simulink model "HQEV_MiL_20160830_integrate"  (Simulink 8.3)
settings: Solver=FixedStepDiscrete  StartTime=0.0  StopTime=inf  FixedStep=0.01  RelTol=1e-3
PostLoadFcn:
  | , if any(exist('dsrtsu_mdlpostloadfcn', 'file') == [2, 3, 6]), try dsrtsu_mdlpostloadfcn('Execute', bdroot); catch fprintf('Error in PostLoadFcn (dsrtsu_mdlpostloadfcn) for model "%s":\n %s\n', bdroot, lasterr); end, end,
values from neighbouring files (symbols this model uses):
  Bat_C_Ah = 36    [parameter_V1.mat]
  Bat_ocv_xIndex = [5 10 20 30 40 50 60 70 80 90 95]    [parameter_V1.mat]
  Bat_ocv_z = [329 332 340 345 347 351 358 372 377 386 391]    [parameter_V1.mat]
  Bat_R_ohm_z = [4.41 3.46 1.57 1.07 0.76 0.63 0.55 0.44 0.41 0.4 0.4 3.14 ... (66 elements, 11x6)]    [parameter_V1.mat]
  Bat_SOC_Init = 90    [parameter_V1.mat]
  Env_hum_pct_Ambient = 30    [parameter_V1.mat]
  Env_Slope_deg = 0    [parameter_V1.mat]
  Env_Temp_degC_Ambient = 25    [parameter_V1.mat]
  Env_v_kmph_HWind = 0    [parameter_V1.mat]
  Reducer_F_i = 7.23    [parameter_V1.mat]
  Reducer_R_i = 7.23    [parameter_V1.mat]
  Veh =     [parameter_V1.mat]
  Veh_A_m2_Fr = 2.246    [parameter_V1.mat]
  Veh_F_Brake =     [parameter_V1.mat]
  Veh_fac_AirDrag = 0.326    [parameter_V1.mat]
  Veh_fac_WhDragFrict_0 = 0.011    [parameter_V1.mat]
  Veh_g_mps2_C = 9.81    [parameter_V1.mat]
  Veh_GainBrake =     [parameter_V1.mat]
  Veh_h_m_COGHigh = 0.5    [parameter_V1.mat]
  Veh_J_kgm2_Wh = 1.3635    [parameter_V1.mat]
  Veh_L_m_AxlBas = 2.63    [parameter_V1.mat]
  Veh_M_kg = 1427    [parameter_V1.mat]
  Veh_mu_Brake = 0.4    [parameter_V1.mat]
  Veh_mu_Tyre =     [parameter_V1.mat]
  Veh_num_FrictPair = 8    [parameter_V1.mat]
  Veh_pct_Brk = 70    [parameter_V1.mat]
  Veh_r_dyn =     [parameter_V1.mat]
  Veh_r_m_BrkDisk = 0.136    [parameter_V1.mat]
  Veh_rho_kgpm3_Air = 1.2258    [parameter_V1.mat]
undefined symbols (not defined in the file or in its folder): DiscIntNeverNeededParam, p_bool_False_M, p_bool_True_M
libraries: BaseOperationLib_Browser x38, simulink x9, DTQC_lib x1, ERR_lib x1, MQM_lib x1, PTCL_lib x1, PUD_lib x1, TQD_lib x1, TQR_lib x1, VMM_lib x1, ACCA_lib x1, BBCA_lib x1
(part 8 of 15)

== system HQEV_MiL_20160830_integrate/MiL/Test_Integration/DCDC/DCDC/DCDC/Electric_Manage ==
  DCDC_enable : Inport
  V_out_req : Inport  Port=2
  Battery_Voltage : Inport  Port=3
  IO_In1 : Inport  Port=4
  Constant1 : Constant  Value=0
  Constant2 : Constant  Value=400
  Constant4 : Constant  Value=0.85
  DCDCStatus : Subsystem
  Divide : Product  Inputs=*/
  Divide1 : Product  Inputs=*/
  Multiport Switch : MultiPortSwitch  DataPortOrder=Zero-based contiguous  Inputs=2  zeroidx=on
  P/U : Product  Inputs=*/
  Saturation : Saturate  UpperLimit=30  LowerLimit=10
  Saturation1 : Saturate  UpperLimit=500  LowerLimit=200
  DCDC_Status : Outport
  DCDC_pwr_Output : Outport  Port=2
  DCDC_pwr_Input : Outport  Port=3
  DCDC_I_Input : Outport  Port=4
  DCDC_U_Input : Outport  Port=5
  DCDC_I_Output : Outport  Port=6
  DCDC_U_Output : Outport  Port=7
  wires:
  V_out_req/1 -> Saturation/1
  P/U/1 -> DCDC_I_Output/1
  DCDC_enable/1 -> Multiport Switch/1, DCDCStatus/1(DCDC_Enable)
  Multiport Switch/1 -> P/U/1, Divide/1, DCDC_pwr_Output/1
  Constant1/1 -> Multiport Switch/2
  Saturation/1 -> P/U/2, DCDC_U_Output/1
  Constant4/1 -> Divide/2
  Battery_Voltage/1 -> Saturation1/1
  Saturation1/1 -> Divide1/2, DCDC_U_Input/1
  Divide1/1 -> DCDC_I_Input/1
  DCDCStatus/1(StatusDCDC) -> DCDC_Status/1
  Divide/1 -> Divide1/1, DCDC_pwr_Input/1
  Constant2/1 -> Multiport Switch/3
  IO_In1/1 -> DCDCStatus/2(IO_In1)

== system HQEV_MiL_20160830_integrate/MiL/Test_Integration/DCDC/DCDC/Output/Checksum_DCDC1 ==
  In1 : Inport
  Constant : Constant  Value=0
  Terminator : Terminator
  Checksum_DCDC1 : Outport
  wires:
  Constant/1 -> Checksum_DCDC1/1
  In1/1 -> Terminator/1

== system HQEV_MiL_20160830_integrate/MiL/Test_Integration/DCDC/DCDC/Output/DCDCLoss ==
  In1 : Inport
  Bus Selector : BusSelector  OutputSignals=signal2.DCDC_Input_Power
  Constant : Constant  Value=0.15
  Product : Product  RndMeth=Zero
  pwr_DCDCLoss : Outport
  wires:
  Bus Selector/1 -> Product/1  "<DCDC_Input_Power>"
  In1/1 -> Bus Selector/1
  Constant/1 -> Product/2
  Product/1 -> pwr_DCDCLoss/1

== system HQEV_MiL_20160830_integrate/MiL/Test_Integration/DCDC/DCDC/Output/DCDC_InputCurrent ==
  In1 : Inport
  Bus Selector : BusSelector  OutputSignals=signal2.DCDC_Input_Current
  DCDC_in_Current : Outport
  wires:
  In1/1 -> Bus Selector/1
  Bus Selector/1 -> DCDC_in_Current/1  "<DCDC_Input_Current>"

== system HQEV_MiL_20160830_integrate/MiL/Test_Integration/DCDC/DCDC/Output/DCDC_InputVoltage ==
  In1 : Inport
  Bus Selector : BusSelector  OutputSignals=signal2.DCDC_Input_Voltage
  DCDC_Input_Voltage : Outport
  wires:
  In1/1 -> Bus Selector/1
  Bus Selector/1 -> DCDC_Input_Voltage/1  "<DCDC_Input_Voltage>"

== system HQEV_MiL_20160830_integrate/MiL/Test_Integration/DCDC/DCDC/Output/DCDC_Input_Powr ==
  In1 : Inport
  Bus Selector : BusSelector  OutputSignals=signal2.DCDC_Input_Power
  DCDC_Input_Power : Outport
  wires:
  In1/1 -> Bus Selector/1
  Bus Selector/1 -> DCDC_Input_Power/1  "<DCDC_Input_Power>"

== system HQEV_MiL_20160830_integrate/MiL/Test_Integration/DCDC/DCDC/Output/DCDC_OutputCurrent ==
  In : Inport
  Bus Selector : BusSelector  OutputSignals=signal2.DCDC_Output_Current
  DCDC_Output_Current : Outport
  wires:
  Bus Selector/1 -> DCDC_Output_Current/1  "<DCDC_Output_Current>"
  In/1 -> Bus Selector/1

== system HQEV_MiL_20160830_integrate/MiL/Test_Integration/DCDC/DCDC/Output/DCDC_OutputVoltage ==
  In1 : Inport
  Bus Selector : BusSelector  OutputSignals=signal2.DCDC_Output_Voltage
  DCDC_Output_Voltage : Outport
  wires:
  In1/1 -> Bus Selector/1
  Bus Selector/1 -> DCDC_Output_Voltage/1  "<DCDC_Output_Voltage>"

== system HQEV_MiL_20160830_integrate/MiL/Test_Integration/DCDC/DCDC/Output/DCDC_Status ==
  In1 : Inport
  Bus Selector : BusSelector  OutputSignals=signal2.DCDC_Status
  DCDC_Status : Outport
  wires:
  In1/1 -> Bus Selector/1
  Bus Selector/1 -> DCDC_Status/1  "<DCDC_Status>"

== system HQEV_MiL_20160830_integrate/MiL/Test_Integration/DCDC/DCDC/Output/DCDC_Temperature ==
  Constant : Constant  Value=30
  DCDC_Temperature : Outport
  wires:
  Constant/1 -> DCDC_Temperature/1

== system HQEV_MiL_20160830_integrate/MiL/Test_Integration/DCDC/DCDC/Output/LiveCounter_DCDC_1 ==
  In1 : Inport
  Constant : Constant  Value=0
  Terminator : Terminator
  LiveCounter_DCDC1 : Outport
  wires:
  In1/1 -> Terminator/1
  Constant/1 -> LiveCounter_DCDC1/1

== system HQEV_MiL_20160830_integrate/MiL/Test_Integration/Driver/Driver/Control_Panel/ACButton ==
  note: 0 no press
      | 1      press
  IO_IN : Inport
  Bus Selector : BusSelector  OutputSignals=AC_Button
  out : Outport
  wires:
  Bus Selector/1 -> out/1  "<AC_Button>"
  IO_IN/1 -> Bus Selector/1

== system HQEV_MiL_20160830_integrate/MiL/Test_Integration/Driver/Driver/Control_Panel/ACC_Cruise_Button ==
  IO_IN : Inport
  Bus Selector : BusSelector  OutputSignals=ACCCruseInput
  Cancel_2 : Constant  Value=1000
  Error : Constant  Value=10000
  Headway_4 : Constant  Value=3200
  MainOff_0 : Constant  Value=5000
  MainOn_1 : Constant  Value=4500
  Multiport Switch : MultiPortSwitch  DataPortOrder=Zero-based contiguous  Inputs=7  zeroidx=on
  Resume_5 : Constant  Value=3900
  Set_3 : Constant  Value=2300
  out : Outport
  wires:
  IO_IN/1 -> Bus Selector/1
  Bus Selector/1 -> Multiport Switch/1  "<ACCCruseInput>"
  MainOff_0/1 -> Multiport Switch/2
  MainOn_1/1 -> Multiport Switch/3
  Cancel_2/1 -> Multiport Switch/4
  Set_3/1 -> Multiport Switch/5
  Headway_4/1 -> Multiport Switch/6
  Resume_5/1 -> Multiport Switch/7
  Multiport Switch/1 -> out/1
  Error/1 -> Multiport Switch/8

== system HQEV_MiL_20160830_integrate/MiL/Test_Integration/Driver/Driver/Control_Panel/ACStation_U ==
  Constant : Constant  Value=220
  out : Outport
  wires:
  Constant/1 -> out/1

== system HQEV_MiL_20160830_integrate/MiL/Test_Integration/Driver/Driver/Control_Panel/CP ==
  Constant : Constant  Value=0
  out : Outport
  wires:
  Constant/1 -> out/1

== system HQEV_MiL_20160830_integrate/MiL/Test_Integration/Driver/Driver/Control_Panel/EGSM_ECOSButton ==
  note: 0 no press
      | 1      press
  Constant : Constant  Value=0
  out : Outport
  wires:
  Constant/1 -> out/1

== system HQEV_MiL_20160830_integrate/MiL/Test_Integration/Driver/Driver/Control_Panel/EGSM_KnobPosition ==
  note: 0  center
      | 1        up
      | 3   down
  Constant : Constant  Value=0
  out : Outport
  wires:
  Constant/1 -> out/1

== system HQEV_MiL_20160830_integrate/MiL/Test_Integration/Driver/Driver/Control_Panel/EGSM_ParkButton ==
  note: 0 no press
      | 1      press
  Constant : Constant  Value=0
  out : Outport
  wires:
  Constant/1 -> out/1

== system HQEV_MiL_20160830_integrate/MiL/Test_Integration/Driver/Driver/Control_Panel/EGSM_SecurityButton ==
  note: 0 no press
      | 1      press
  Constant : Constant  Value=0
  out : Outport
  wires:
  Constant/1 -> out/1

== system HQEV_MiL_20160830_integrate/MiL/Test_Integration/Driver/Driver/Control_Panel/FastCharge ==
  IO_IN : Inport
  Bus Selector : BusSelector  OutputSignals=ChargeCheck
  ChargeFault : Constant  Value=220
  FastCharge : Constant  Value=1020
  Multiport Switch : MultiPortSwitch  DataPortOrder=Zero-based contiguous  Inputs=4  zeroidx=on
  NoCharge : Constant  Value=0
  Saturation : Saturate  UpperLimit=3  LowerLimit=0
  SlowCharge : Constant  Value=270
  out : Outport
  wires:
  Bus Selector/1 -> Saturation/1  "<ChargeCheck>"
  IO_IN/1 -> Bus Selector/1
  Multiport Switch/1 -> out/1
  NoCharge/1 -> Multiport Switch/2
  ChargeFault/1 -> Multiport Switch/5
  Saturation/1 -> Multiport Switch/1
  SlowCharge/1 -> Multiport Switch/4
  FastCharge/1 -> Multiport Switch/3

== system HQEV_MiL_20160830_integrate/MiL/Test_Integration/Driver/Driver/Control_Panel/InterlockA ==
  IO_IN : Inport
  Bus Selector : BusSelector  OutputSignals=interlockA
  Compare To Constant : simulink/Logic and Bit Operations/Compare To Constant  SystemSampleTime=-1  relop===  const=0  LogicOutDataTypeMode=boolean
  Init : Constant  Value=2500
  Switch : Switch  Criteria=u2 > Threshold
  out : Outport
  wires:
  IO_IN/1 -> Bus Selector/1
  Bus Selector/1 -> Switch/3, Compare To Constant/1  "<interlockA>"
  Compare To Constant/1 -> Switch/2
  Init/1 -> Switch/1
  Switch/1 -> out/1

== system HQEV_MiL_20160830_integrate/MiL/Test_Integration/Driver/Driver/Control_Panel/InterlockB ==
  IO_IN : Inport
  Bus Selector : BusSelector  OutputSignals=interlockB
  Compare To Constant : simulink/Logic and Bit Operations/Compare To Constant  SystemSampleTime=-1  relop===  const=0  LogicOutDataTypeMode=boolean
  Init : Constant  Value=2500
  Switch : Switch  Criteria=u2 > Threshold
  out : Outport
  wires:
  IO_IN/1 -> Bus Selector/1
  Compare To Constant/1 -> Switch/2
  Init/1 -> Switch/1
  Bus Selector/1 -> Switch/3, Compare To Constant/1  "<interlockB>"
  Switch/1 -> out/1

== system HQEV_MiL_20160830_integrate/MiL/Test_Integration/Driver/Driver/Control_Panel/KeyONState ==
  IO_IN : Inport
  Bus Selector : BusSelector  OutputSignals=KeyOn
  out : Outport
  wires:
  Bus Selector/1 -> out/1  "<KeyOn>"
  IO_IN/1 -> Bus Selector/1

== system HQEV_MiL_20160830_integrate/MiL/Test_Integration/Driver/Driver/Control_Panel/KeyStartState ==
  IO_IN : Inport
  Bus Selector : BusSelector  OutputSignals=KeyStart
  out : Outport
  wires:
  Bus Selector/1 -> out/1  "<KeyStart>"
  IO_IN/1 -> Bus Selector/1

== system HQEV_MiL_20160830_integrate/MiL/Test_Integration/Driver/Driver/Control_Panel/LeverPosition ==
  note: 0--Center
      | 1--up
      | 2--down
      | 3--up up
      | 4--down down
  IO_IN : Inport
  Bus Selector : BusSelector  OutputSignals=ShiftLeverInput
  Center : Constant  Value=0
  Down : Constant  Value=2
  DownDown : Constant  Value=4
  Multiport Switch : MultiPortSwitch  DataPortOrder=Zero-based contiguous  Inputs=5  zeroidx=on
  Saturation : Saturate  UpperLimit=4  LowerLimit=0
  Up : Constant
  UpUp : Constant  Value=3
  out : Outport
  wires:
  Multiport Switch/1 -> out/1
  IO_IN/1 -> Bus Selector/1
  Bus Selector/1 -> Saturation/1  "<ShiftLeverInput>"
  Center/1 -> Multiport Switch/2
  Up/1 -> Multiport Switch/3
  Down/1 -> Multiport Switch/4
  UpUp/1 -> Multiport Switch/5
  DownDown/1 -> Multiport Switch/6
  Saturation/1 -> Multiport Switch/1

== system HQEV_MiL_20160830_integrate/MiL/Test_Integration/Driver/Driver/Control_Panel/RunSignal ==
  Constant : Constant  Value=0
  out : Outport
  wires:
  Constant/1 -> out/1

== system HQEV_MiL_20160830_integrate/MiL/Test_Integration/Driver/Driver/Driver_AutoPedal/CTRL AccPed ==
  v_set [km/h] : Inport
  v_Veh [km/h] : Inport  Port=2
  Brake [%] : Inport  Port=3
  Brake off : Subsystem  mask(Compare To Constant){relop=<=, const=eps, LogicOutDataTypeMode=uint8, ZeroCross=off}
      mask prompts: relop "Operator:"; const "Constant value:"; LogicOutDataTypeMode "Output data type mode:"; ZeroCross "Enable zero crossing detection"
      mask help: Determine how a signal compares to a constant.
      mask init:
      | blkName = gcb;
      | 
      | if strcmp(get_param(gcbh,'LogicOutDataTypeMode'),'boolean')
      | 	setValue = 'Boolean';
      | else
      | 	setValue = 'Specify via dialog';
      | end
      | 
      | set_param([blkName,'/Compare'],'relop',relop, ...
      | 	'LogicOutDataTypeMode', setValue, 'ZeroCross', ZeroCross);
      | 
      | str = [relop,' C']; %default
      | 
      | const_str = get_param(blkName, 'const');
      | 
      | if isempty(strfind(const_str, ' ')) && isempty(strfind(const_str, ','))
      |     % scalar or single expression
      |     if isempty(str2num(const_str))
      |         %expression
      |         str = [relop, ' ', const_str];
      |     elseif length(const) == 1
      |         str = [relop,' ',num2str(double(const))];
      |     end
      | end
      mask TypeOptions relop: == | ~= | < | <= | >= | >
      mask TypeOptions LogicOutDataTypeMode: uint8 | boolean
      mask Callback ZeroCross: sl('zeroCrossEnable', gcbh);
      mask Display: disp(str)
  Constant : Constant  Value=0
  Constant4 : Constant  Value=0
  Discrete-Time Integrator : DiscreteIntegrator  ExternalReset=rising  InitialConditionSource=external  SampleTime=-1  LimitOutput=on  UpperSaturationLimit=50  LowerSaturationLimit=-20  ICPrevOutput=DiscIntNeverNeededParam  ICPrevScaledInput=DiscIntNeverNeededParam
  I_value : Gain  Gain=0.1  SaturateOnIntegerOverflow=on  OutDataTypeStr=Inherit: Same as input  ParamDataTypeStr=Inherit: Same as input
  P_value : Gain  Gain=0.1  SaturateOnIntegerOverflow=on  OutDataTypeStr=Inherit: Same as input  ParamDataTypeStr=Inherit: Same as input
  Reset : Subsystem
  Saturation : Saturate  UpperLimit=100  LowerLimit=0
  Subsystem : Subsystem
  Sum : Sum  Inputs=|++  SaturateOnIntegerOverflow=on  InputSameDT=on  OutDataTypeStr=Inherit: Same as first input
  Switch3 : Switch  Criteria=u2 ~= 0  Threshold=0.5
  Sig_AccPed [%] : Outport
  wires:
  Subsystem/1(error) -> I_value/1, Reset/1(v_error), P_value/1
  Constant/1 -> Discrete-Time Integrator/3
  I_value/1 -> Discrete-Time Integrator/1
  Reset/1(reset) -> Discrete-Time Integrator/2
  P_value/1 -> Sum/1  "P-Anteil"
  Discrete-Time Integrator/1 -> Sum/2  "I-Anteil"
  Saturation/1 -> Switch3/1  "Gaspedal"
  Brake off/1(y) -> Switch3/2
  Sum/1 -> Saturation/1  "result"
  Constant4/1 -> Switch3/3
  Switch3/1 -> Sig_AccPed [%]/1
  Brake [%]/1 -> Reset/3(Brake [%]), Brake off/1(u)
  v_set [km/h]/1 -> Subsystem/1(v_Set), Reset/2(v_Set)
  v_Veh [km/h]/1 -> Subsystem/2(v_Veh)

== system HQEV_MiL_20160830_integrate/MiL/Test_Integration/Driver/Driver/Driver_AutoPedal/CTRL BrakePed ==
  v_set [km/h] : Inport
  v_Veh [km/h] : Inport  Port=2
  Bus Creator : BusCreator  Inputs=6
  Bus Selector : BusSelector  OutputSignals=v_set,v_Veh
  Bus Selector1 : BusSelector  OutputSignals=delta_v_set,v_error
  Bus Selector2 : BusSelector  OutputSignals=delta_v_set,v_error,v_Veh,Brake,Brake_set
  Bus Selector3 : BusSelector  OutputSignals=v_error
  Bus Selector4 : BusSelector  OutputSignals=v_set
  Constant : Constant  Value=50
  PI-Regler : Subsystem
  Reset_Block : Subsystem
  S-R Flip-Flop : Subsystem  mask(SRFlipFlop){initial_condition=0}
      mask prompts: initial_condition "Initial condition (state of Q):"
      mask help: S-R Flip-Flop Block
      mask Help:
      | The S-R flip-flop also known as a set-reset flip-flop. This implementation
      | is modeled after an S-R flip-flop constructed using NOR gates. The
      | truth table for this block is:
      | <pre>
      |  S  R   Q  !Q
      |  ----------------
      |  1  0   1  0
      |  0  0   1  0  (after S == 1, R == 0)
      |  0  1   0  1
      |  0  0   0  1  (after S == 0, R == 1)
      |  1  1   0  0
      | </pre>
      | 
      | In an S-R flip-flop that is implemented with NOR gates, when a 1 is
      | applied to both the set and reset inputs, both outputs go to 0. Technically,
      | this state is undefined and is usually avoided. Note, if the flip-flop is
      | implemented with NAND gates, when a 0 is applied to both inputs, both outputs
      | go to 0 and when a 1 is applied to both inputs, the output depends on
      | the previous state of the flip-flop (previous value of Q).
  Set_Block : Subsystem
  Switch : Switch  Criteria=u2 > Threshold
  Terminator : Terminator
  Unit Delay1 : UnitDelay  SampleTime=-1
  velocoty : Subsystem
  "Brake[%] " : Outport
  wires:
  PI-Regler/1(Result) -> Unit Delay1/1, Switch/1
  Reset_Block/1(Brake_Reset) -> S-R Flip-Flop/2(R)
  S-R Flip-Flop/2(!Q) -> Terminator/1
  S-R Flip-Flop/1(Q) -> PI-Regler/Enable
  Set_Block/1(Brake_set) -> S-R Flip-Flop/1(S), Bus Creator/3  "Brake_set"
  v_Veh [km/h]/1 -> Bus Creator/6  "v_Veh"
  v_set [km/h]/1 -> Bus Creator/5  "v_set"
  velocoty/1(delta_v_set) -> Bus Creator/1  "delta_v_set"
  velocoty/2(v_error) -> Bus Creator/2  "v_error"
  Unit Delay1/1 -> Bus Creator/4  "Brake"
  Bus Creator/1 -> Bus Selector/1, Bus Selector1/1, Bus Selector2/1, Bus Selector3/1, Bus Selector4/1
  Bus Selector/1 -> velocoty/1(v_set [km/h])  "<v_set>"
  Bus Selector/2 -> velocoty/2(v_Veh [km/h])  "<v_Veh>"
  Bus Selector1/1 -> Set_Block/1(delta_v_set)  "<delta_v_set>"
  Bus Selector1/2 -> Set_Block/2(v_error)  "<v_error>"
  Bus Selector2/1 -> Reset_Block/1(delta_v_set)  "<delta_v_set>"
  Bus Selector2/2 -> Reset_Block/2(v_error)  "<v_error>"
  Bus Selector2/3 -> Reset_Block/3(v_Veh)  "<v_Veh>"
  Bus Selector2/4 -> Reset_Block/4(Brake)  "<Brake>"
  Bus Selector2/5 -> Reset_Block/5(Brake_Set)  "<Brake_set>"
  Bus Selector3/1 -> PI-Regler/1(error)  "<v_error>"
  Bus Selector4/1 -> Switch/2  "<v_set>"
  Switch/1 -> "Brake[%] "/1
  Constant/1 -> Switch/3

== system HQEV_MiL_20160830_integrate/MiL/Test_Integration/Driver/Driver/Driver_AutoPedal/Stop_Indicator ==
  v_set : Inport
  Logical Operator : Logic  AllPortsSameDT=off  OutDataTypeStr=boolean
  Logical Operator1 : Logic  AllPortsSameDT=off  OutDataTypeStr=boolean
  Logical Operator2 : Logic  Operator=OR  AllPortsSameDT=off  OutDataTypeStr=boolean
  v_Set<0 : Subsystem  mask(Compare To Constant){relop=>=, const=-eps, LogicOutDataTypeMode=uint8, ZeroCross=off}
      mask prompts: relop "Operator:"; const "Constant value:"; LogicOutDataTypeMode "Output data type mode:"; ZeroCross "Enable zero crossing detection"
      mask help: Determine how a signal compares to a constant.
      mask init: same as HQEV_MiL_20160830_integrate/MiL/Test_Integration/Driver/Driver/Driver_AutoPedal/CTRL AccPed/Brake off
      mask TypeOptions relop: == | ~= | < | <= | >= | >
      mask TypeOptions LogicOutDataTypeMode: uint8 | boolean
      mask Callback ZeroCross: sl('zeroCrossEnable', gcbh);
      mask Display: disp(str)
  v_Set==1 : Subsystem  mask(Compare To Constant){relop=<, const=0, LogicOutDataTypeMode=uint8, ZeroCross=off}
      mask prompts: relop "Operator:"; const "Constant value:"; LogicOutDataTypeMode "Output data type mode:"; ZeroCross "Enable zero crossing detection"
      mask help: Determine how a signal compares to a constant.
      mask init: same as HQEV_MiL_20160830_integrate/MiL/Test_Integration/Driver/Driver/Driver_AutoPedal/CTRL AccPed/Brake off
      mask TypeOptions relop: == | ~= | < | <= | >= | >
      mask TypeOptions LogicOutDataTypeMode: uint8 | boolean
      mask Callback ZeroCross: sl('zeroCrossEnable', gcbh);
      mask Display: disp(str)
  v_Set==2 : Subsystem  mask(Compare To Constant){relop=>=, const=0, LogicOutDataTypeMode=uint8, ZeroCross=off}
      mask prompts: relop "Operator:"; const "Constant value:"; LogicOutDataTypeMode "Output data type mode:"; ZeroCross "Enable zero crossing detection"
      mask help: Determine how a signal compares to a constant.
      mask init: same as HQEV_MiL_20160830_integrate/MiL/Test_Integration/Driver/Driver/Driver_AutoPedal/CTRL AccPed/Brake off
      mask TypeOptions relop: == | ~= | < | <= | >= | >
      mask TypeOptions LogicOutDataTypeMode: uint8 | boolean
      mask Callback ZeroCross: sl('zeroCrossEnable', gcbh);
      mask Display: disp(str)
  "v_Set>=0 " : Subsystem  mask(Compare To Constant){relop=<=, const=eps, LogicOutDataTypeMode=uint8, ZeroCross=off}
      mask prompts: relop "Operator:"; const "Constant value:"; LogicOutDataTypeMode "Output data type mode:"; ZeroCross "Enable zero crossing detection"
      mask help: Determine how a signal compares to a constant.
      mask init: same as HQEV_MiL_20160830_integrate/MiL/Test_Integration/Driver/Driver/Driver_AutoPedal/CTRL AccPed/Brake off
      mask TypeOptions relop: == | ~= | < | <= | >= | >
      mask TypeOptions LogicOutDataTypeMode: uint8 | boolean
      mask Callback ZeroCross: sl('zeroCrossEnable', gcbh);
      mask Display: disp(str)
  stop : Outport
  wires:
  v_set/1 -> v_Set<0/1(u), v_Set==1/1(u), "v_Set>=0 "/1(u), v_Set==2/1(u)
  v_Set<0/1(y) -> Logical Operator/1
  v_Set==1/1(y) -> Logical Operator/2
  "v_Set>=0 "/1(y) -> Logical Operator1/1
  v_Set==2/1(y) -> Logical Operator1/2
  Logical Operator/1 -> Logical Operator2/1
  Logical Operator1/1 -> Logical Operator2/2
  Logical Operator2/1 -> stop/1

== system HQEV_MiL_20160830_integrate/MiL/Test_Integration/EPS/EPS/Subsystem2/Subsystem ==
  Constant1 : Constant  Value=0
  EPSErrorStatus : Outport
  wires:
  Constant1/1 -> EPSErrorStatus/1

== system HQEV_MiL_20160830_integrate/MiL/Test_Integration/EPS/EPS/Subsystem2/Subsystem1 ==
  Constant : Constant  Value=0
  SteeringWheelAngleStatus : Outport
  wires:
  Constant/1 -> SteeringWheelAngleStatus/1

== system HQEV_MiL_20160830_integrate/MiL/Test_Integration/Epark/Subsystem/Epark/Epark_Process ==
  In3 : Inport
  EPark_Process : Stateflow chart  TreatAsAtomicUnit=on
  st_pParkRequest_M : Constant
  st_pUnparkRequest_M : Constant  Value=2
  ParkLock : Outport
  ParkSensor : Outport  Port=2
  DriveSensor : Outport  Port=3
  wires:
  EPark_Process/1(st_ParkLoceState) -> ParkLock/1
  EPark_Process/2(bool_ParkSensor) -> ParkSensor/1
  EPark_Process/3(bool_DriveSensor) -> DriveSensor/1
  st_pParkRequest_M/1 -> EPark_Process/2(st_pParkRequest_M)
  st_pUnparkRequest_M/1 -> EPark_Process/3(st_pUnparkRequest_M)

== system HQEV_MiL_20160830_integrate/MiL/Test_Integration/Epark/Subsystem/Epark/Subsystem ==
  Constant : Constant  Value=0
  ePARK_MOTOR_OPEN_CKT : Outport
  wires:
  Constant/1 -> ePARK_MOTOR_OPEN_CKT/1

== system HQEV_MiL_20160830_integrate/MiL/Test_Integration/Epark/Subsystem/Epark/Subsystem1 ==
  Constant1 : Constant  Value=0
  ePARK_MOTOR_JAMMED_PARK : Outport
  wires:
  Constant1/1 -> ePARK_MOTOR_JAMMED_PARK/1

== system HQEV_MiL_20160830_integrate/MiL/Test_Integration/Epark/Subsystem/Epark/Subsystem2 ==
  Constant2 : Constant
  ePARK_MOTOR_JAMMED_UNPARK : Outport
  wires:
  Constant2/1 -> ePARK_MOTOR_JAMMED_UNPARK/1

== system HQEV_MiL_20160830_integrate/MiL/Test_Integration/Epark/Subsystem/Epark/Subsystem3 ==
  Constant3 : Constant  Value=0
  ePARK_MOTOR_JAMMED_MIDDL : Outport
  wires:
  Constant3/1 -> ePARK_MOTOR_JAMMED_MIDDL/1

== system HQEV_MiL_20160830_integrate/MiL/Test_Integration/Epark/Subsystem/Epark/Subsystem4 ==
  Constant4 : Constant  Value=0
  ePARK_HALL_SENSOR_INVALID : Outport
  wires:
  Constant4/1 -> ePARK_HALL_SENSOR_INVALID/1

== system HQEV_MiL_20160830_integrate/MiL/Test_Integration/Epark/Subsystem/Epark/Subsystem5 ==
  Constant5 : Constant  Value=0
  ePARK_LOST_COMM_VCU : Outport
  wires:
  Constant5/1 -> ePARK_LOST_COMM_VCU/1

== system HQEV_MiL_20160830_integrate/MiL/Test_Integration/Epark/Subsystem/Epark/Subsystem6 ==
  Constant6 : Constant  Value=0
  ePARK_CAN_ERR : Outport
  wires:
  Constant6/1 -> ePARK_CAN_ERR/1

== system HQEV_MiL_20160830_integrate/MiL/Test_Integration/HCU/HCU/HCU/EVManager ==
  RTEIn : Inport
  evm_core : Subsystem
  hw_algo : Subsystem
  hw_post : Subsystem
  hw_prep : Subsystem
  RTEOut : Outport
  tag scope: evm_core=global
  wires:
  evm_core/1(Bus_evm_core) -> hw_post/1(Bus_evm_core), hw_algo/1(Bus_evm_core), [evm_core]
  hw_algo/1(Bus_hw_algo) -> hw_post/2(Bus_hw_algo), evm_core/2(Bus_hw_algo)
  hw_prep/1(Bus_hw_prep) -> hw_post/3(Bus_hw_prep), hw_algo/2(Bus_hw_prep), evm_core/1(Bus_hw_prep)
  hw_post/1(Bus_RTE_out) -> RTEOut/1
  RTEIn/1 -> hw_prep/1(Bus_RTE_in)

== system HQEV_MiL_20160830_integrate/MiL/Test_Integration/MCU_FF/MCU/MCU/GSD ==
  In1 : Inport
  function : TriggerPort  TriggerType=function-call
  Bus Creator : BusCreator  Inputs=14
  Subsystem : Subsystem
  Out1 : Outport
  wires:
  Subsystem/13(EM_trq_req) -> Bus Creator/13  "EM_trq_req"
  Subsystem/12(PWM_Status) -> Bus Creator/12  "PWM_Status"
  Subsystem/11(MCU1_CoolingRequest) -> Bus Creator/11  "MCU1_CoolingRequest"
  Subsystem/10(MCU1_CalTMTorque) -> Bus Creator/10  "MCU1_CalTMTorque"
  Subsystem/9(MCU1_TM MAGTorque) -> Bus Creator/9  "MCU1_TMMAGTorque"
  Subsystem/8(MCU1_TM MAMTorque) -> Bus Creator/8  "MCU1_TMMAMTorque"
  Subsystem/7(MCU1_TMErrorStatus) -> Bus Creator/7  "MCU1_TMErrorStatus"
  Subsystem/6(MCU1_TMStatus) -> Bus Creator/6  "MCU1_TMStatus"
  Subsystem/5(MCU1_MCU1 PrechargeAllow) -> Bus Creator/5  "MCU1_MCU1 PrechargeAllow"
  Subsystem/4(MCU1_ActualTMTorqueValid) -> Bus Creator/4  "MCU1_ActualTMTorqueValid"
  Subsystem/3(MCU1_TMCapacitanceVoltage) -> Bus Creator/3  "MCU1_TMCapacitanceVoltage"
  Subsystem/2(MCU1_ActTMTorque) -> Bus Creator/2  "MCU1_ActTMTorque"
  Subsystem/1(MCU1_TMSpeed) -> Bus Creator/1  "MCU1_TMSpeed"
  Bus Creator/1 -> Out1/1
  In1/1 -> Subsystem/1(In1)
  Subsystem/14(bool_MCUPwrDwnAllow) -> Bus Creator/14  "bool_MCUPwrDownAllow"

== system HQEV_MiL_20160830_integrate/MiL/Test_Integration/MCU_FF/MCU/MCU/Init ==
  In1 : Inport
  function : TriggerPort  TriggerType=function-call
  Bus Creator : BusCreator  Inputs=14
  Subsystem : Subsystem
  Out1 : Outport
  wires:
  Bus Creator/1 -> Out1/1
  Subsystem/13(EM_trq_req) -> Bus Creator/13  "EM_trq_req"
  Subsystem/12(PWM_Status) -> Bus Creator/12  "PWM_Status"
  Subsystem/11(MCU1_CoolingRequest) -> Bus Creator/11  "MCU1_CoolingRequest"
  Subsystem/10(MCU1_CalTMTorque) -> Bus Creator/10  "MCU1_CalTMTorque"
  Subsystem/9(MCU1_TM MAGTorque) -> Bus Creator/9  "MCU1_TMMAGTorque"
  Subsystem/8(MCU1_TM MAMTorque) -> Bus Creator/8  "MCU1_TMMAMTorque"
  Subsystem/7(MCU1_TMErrorStatus) -> Bus Creator/7  "MCU1_TMErrorStatus"
  Subsystem/6(MCU1_TMStatus) -> Bus Creator/6  "MCU1_TMStatus"
  Subsystem/5(MCU1_MCU1PrechargeAllow) -> Bus Creator/5  "MCU1_MCU1 PrechargeAllow"
  Subsystem/4(MCU1_ActualTMTorqueValid) -> Bus Creator/4  "MCU1_ActualTMTorqueValid"
  Subsystem/3(MCU1_TMCapacitanceVoltage) -> Bus Creator/3  "MCU1_TMCapacitanceVoltage"
  Subsystem/2(MCU1_ActTMTorque) -> Bus Creator/2  "MCU1_ActTMTorque"
  Subsystem/1(MCU1_TMSpeed) -> Bus Creator/1  "MCU1_TMSpeed"
  In1/1 -> Subsystem/1(In1)
  Subsystem/14(bool_MCUPwrDwnAllow) -> Bus Creator/14  "bool_MCUPwrDownAllow"

== system HQEV_MiL_20160830_integrate/MiL/Test_Integration/MCU_FF/MCU/MCU/Invalid ==
  In1 : Inport
  function : TriggerPort  TriggerType=function-call
  Bus Creator : BusCreator  Inputs=14
  Subsystem : Subsystem
  Out1 : Outport
  wires:
  Subsystem/13(EM_trq_req) -> Bus Creator/13  "EM_trq_req"
  Subsystem/12(PWM_Status) -> Bus Creator/12  "PWM_Status"
  Subsystem/11(MCU1_CoolingRequest) -> Bus Creator/11  "MCU1_CoolingRequest"
  Subsystem/10(MCU1_CalTMTorque) -> Bus Creator/10  "MCU1_CalTMTorque"
  Subsystem/9(MCU1_TM MAGTorque) -> Bus Creator/9  "MCU1_TMMAGTorque"
  Subsystem/8(MCU1_TM MAMTorque) -> Bus Creator/8  "MCU1_TMMAMTorque"
  Subsystem/7(MCU1_TMErrorStatus) -> Bus Creator/7  "MCU1_TMErrorStatus"
  Subsystem/6(MCU1_TMStatus) -> Bus Creator/6  "MCU1_TMStatus"
  Subsystem/5(MCU1_MCU1 PrechargeAllow) -> Bus Creator/5  "MCU1_MCU1 PrechargeAllow"
  Subsystem/4(MCU1_ActualTMTorqueValid) -> Bus Creator/4  "MCU1_ActualTMTorqueValid"
  Subsystem/3(MCU1_TMCapacitanceVoltage) -> Bus Creator/3  "MCU1_TMCapacitanceVoltage"
  Subsystem/2(MCU1_ActTMTorque) -> Bus Creator/2  "MCU1_ActTMTorque"
  Subsystem/1(MCU1_TMSpeed) -> Bus Creator/1  "MCU1_TMSpeed"
  Bus Creator/1 -> Out1/1
  In1/1 -> Subsystem/1(In1)
  Subsystem/14(bool_MCUPwrDwnAllow) -> Bus Creator/14  "bool_MCUPwrDownAllow"

== system HQEV_MiL_20160830_integrate/MiL/Test_Integration/MCU_FF/MCU/MCU/Precharge ==
  In1 : Inport
  function : TriggerPort  TriggerType=function-call
  Bus Creator : BusCreator  Inputs=14
  Subsystem : Subsystem
  Out1 : Outport
  wires:
  Bus Creator/1 -> Out1/1
  In1/1 -> Subsystem/1(In1)
  Subsystem/13(EM_trq_req) -> Bus Creator/13  "EM_trq_req"
  Subsystem/12(PWM_Status) -> Bus Creator/12  "PWM_Status"
  Subsystem/11(MCU1_CoolingRequest) -> Bus Creator/11  "MCU1_CoolingRequest"
  Subsystem/10(MCU1_CalTMTorque) -> Bus Creator/10  "MCU1_CalTMTorque"
  Subsystem/9(MCU1_TM MAGTorque) -> Bus Creator/9  "MCU1_TMMAGTorque"
  Subsystem/8(MCU1_TM MAMTorque) -> Bus Creator/8  "MCU1_TMMAMTorque"
  Subsystem/7(MCU1_TMErrorStatus) -> Bus Creator/7  "MCU1_TMErrorStatus"
  Subsystem/6(MCU1_TMStatus) -> Bus Creator/6  "MCU1_TMStatus"
  Subsystem/5(MCU1_MCU1 PrechargeAllow) -> Bus Creator/5  "MCU1_MCU1 PrechargeAllow"
  Subsystem/4(MCU1_ActualTMTorqueValid) -> Bus Creator/4  "MCU1_ActualTMTorqueValid"
  Subsystem/3(MCU1_TMCapacitanceVoltage) -> Bus Creator/3  "MCU1_TMCapacitanceVoltage"
  Subsystem/2(MCU1_ActTMTorque) -> Bus Creator/2  "MCU1_ActTMTorque"
  Subsystem/1(MCU1_TMSpeed) -> Bus Creator/1  "MCU1_TMSpeed"
  Subsystem/14(bool_MCUPwrDwnAllow) -> Bus Creator/14  "bool_MCUPwrDownAllow"

== system HQEV_MiL_20160830_integrate/MiL/Test_Integration/MCU_FF/MCU/MCU/Rapid_Discharge ==
  In1 : Inport
  function : TriggerPort  TriggerType=function-call
  Bus Creator : BusCreator  Inputs=14
  Subsystem : Subsystem
  Out1 : Outport
  wires:
  Subsystem/13(EM_trq_req) -> Bus Creator/13  "EM_trq_req"
  Subsystem/12(PWM_Status) -> Bus Creator/12  "PWM_Status"
  Subsystem/11(MCU1_CoolingRequest) -> Bus Creator/11  "MCU1_CoolingRequest"
  Subsystem/10(MCU1_CalTMTorque) -> Bus Creator/10  "MCU1_CalTMTorque"
  Subsystem/9(MCU1_TM MAGTorque) -> Bus Creator/9  "MCU1_TMMAGTorque"
  Subsystem/8(MCU1_TM MAMTorque) -> Bus Creator/8  "MCU1_TMMAMTorque"
  Subsystem/7(MCU1_TMErrorStatus) -> Bus Creator/7  "MCU1_TMErrorStatus"
  Subsystem/6(MCU1_TMStatus) -> Bus Creator/6  "MCU1_TMStatus"
  Subsystem/5(MCU1_MCU1 PrechargeAllow) -> Bus Creator/5  "MCU1_MCU1 PrechargeAllow"
  Subsystem/4(MCU1_ActualTMTorqueValid) -> Bus Creator/4  "MCU1_ActualTMTorqueValid"
  Subsystem/3(MCU1_TMCapacitanceVoltage) -> Bus Creator/3  "MCU1_TMCapacitanceVoltage"
  Subsystem/2(MCU1_ActTMTorque) -> Bus Creator/2  "MCU1_ActTMTorque"
  Subsystem/1(MCU1_TMSpeed) -> Bus Creator/1  "MCU1_TMSpeed"
  Bus Creator/1 -> Out1/1
  In1/1 -> Subsystem/1(In1)
  Subsystem/14(bool_MCUPwrDwnAllow) -> Bus Creator/14  "bool_MCUPwrDownAllow"

== system HQEV_MiL_20160830_integrate/MiL/Test_Integration/MCU_FF/MCU/MCU/Sleep ==
  In1 : Inport
  function : TriggerPort  TriggerType=function-call
  Bus Creator : BusCreator  Inputs=14
  Subsystem : Subsystem
  Out1 : Outport
  wires:
  Subsystem/13(EM_trq_req) -> Bus Creator/13  "EM_trq_req"
  Subsystem/12(PWM_Status) -> Bus Creator/12  "PWM_Status"
  Subsystem/11(MCU1_CoolingRequest) -> Bus Creator/11  "MCU1_CoolingRequest"
  Subsystem/10(MCU1_CalTMTorque) -> Bus Creator/10  "MCU1_CalTMTorque"
  Subsystem/9(MCU1_TM MAGTorque) -> Bus Creator/9  "MCU1_TMMAGTorque"
  Subsystem/8(MCU1_TM MAMTorque) -> Bus Creator/8  "MCU1_TMMAMTorque"
  Subsystem/7(MCU1_TMErrorStatus) -> Bus Creator/7  "MCU1_TMErrorStatus"
  Subsystem/6(MCU1_TMStatus) -> Bus Creator/6  "MCU1_TMStatus"
  Subsystem/5(MCU1_MCU1 PrechargeAllow) -> Bus Creator/5  "MCU1_MCU1 PrechargeAllow"
  Subsystem/4(MCU1_ActualTMTorqueValid) -> Bus Creator/4  "MCU1_ActualTMTorqueValid"
  Subsystem/3(MCU1_TMCapacitanceVoltage) -> Bus Creator/3  "MCU1_TMCapacitanceVoltage"
  Subsystem/2(MCU1_ActTMTorque) -> Bus Creator/2  "MCU1_ActTMTorque"
  Subsystem/1(MCU1_TMSpeed) -> Bus Creator/1  "MCU1_TMSpeed"
  Bus Creator/1 -> Out1/1
  In1/1 -> Subsystem/1(In1)
  Subsystem/14(bool_MCUPwrDwnAllow) -> Bus Creator/14  "bool_MCUPwrDownAllow"

== system HQEV_MiL_20160830_integrate/MiL/Test_Integration/MCU_FF/MCU/MCU/Standby ==
  In1 : Inport
  function : TriggerPort  TriggerType=function-call
  Bus Creator : BusCreator  Inputs=14
  Subsystem : Subsystem
  Out1 : Outport
  wires:
  In1/1 -> Subsystem/1(In1)
  Subsystem/13(EM_trq_req) -> Bus Creator/13  "EM_trq_req"
  Subsystem/12(PWM_Status) -> Bus Creator/12  "PWM_Status"
  Subsystem/11(MCU1_CoolingRequest) -> Bus Creator/11  "MCU1_CoolingRequest"
  Subsystem/10(MCU1_CalTMTorque) -> Bus Creator/10  "MCU1_CalTMTorque"
  Subsystem/9(MCU1_TM MAGTorque) -> Bus Creator/9  "MCU1_TMMAGTorque"
  Subsystem/8(MCU1_TM MAMTorque) -> Bus Creator/8  "MCU1_TMMAMTorque"
  Subsystem/7(MCU1_TMErrorStatus) -> Bus Creator/7  "MCU1_TMErrorStatus"
  Subsystem/6(MCU1_TMStatus) -> Bus Creator/6  "MCU1_TMStatus"
  Subsystem/5(MCU1_MCU1 PrechargeAllow) -> Bus Creator/5  "MCU1_MCU1 PrechargeAllow"
  Subsystem/4(MCU1_ActualTMTorqueValid) -> Bus Creator/4  "MCU1_ActualTMTorqueValid"
  Subsystem/3(MCU1_TMCapacitanceVoltage) -> Bus Creator/3  "MCU1_TMCapacitanceVoltage"
  Subsystem/2(MCU1_ActTMTorque) -> Bus Creator/2  "MCU1_ActTMTorque"
  Subsystem/1(MCU1_TMSpeed) -> Bus Creator/1  "MCU1_TMSpeed"
  Bus Creator/1 -> Out1/1
  Subsystem/14(bool_MCUPwrDwnAllow) -> Bus Creator/14  "bool_MCUPwrDownAllow"

== system HQEV_MiL_20160830_integrate/MiL/Test_Integration/MCU_FF/MCU/MCU/Stop ==
  In1 : Inport
  function : TriggerPort  TriggerType=function-call
  Bus Creator : BusCreator  Inputs=14
  Subsystem : Subsystem
  Out1 : Outport
  wires:
  In1/1 -> Subsystem/1(In1)
  Subsystem/13(EM_trq_req) -> Bus Creator/13  "EM_trq_req"
  Subsystem/12(PWM_Status) -> Bus Creator/12  "PWM_Status"
  Subsystem/11(MCU1_CoolingRequest) -> Bus Creator/11  "MCU1_CoolingRequest"
  Subsystem/10(MCU1_CalTMTorque) -> Bus Creator/10  "MCU1_CalTMTorque"
  Subsystem/9(MCU1_TM MAGTorque) -> Bus Creator/9  "MCU1_TMMAGTorque"
  Subsystem/8(MCU1_TM MAMTorque) -> Bus Creator/8  "MCU1_TMMAMTorque"
  Subsystem/7(MCU1_TMErrorStatus) -> Bus Creator/7  "MCU1_TMErrorStatus"
  Subsystem/6(MCU1_TMStatus) -> Bus Creator/6  "MCU1_TMStatus"
  Subsystem/5(MCU1_MCU1 PrechargeAllow) -> Bus Creator/5  "MCU1_MCU1 PrechargeAllow"
  Subsystem/4(MCU1_ActualTMTorqueValid) -> Bus Creator/4  "MCU1_ActualTMTorqueValid"
  Subsystem/3(MCU1_TMCapacitanceVoltage) -> Bus Creator/3  "MCU1_TMCapacitanceVoltage"
  Subsystem/2(MCU1_ActTMTorque) -> Bus Creator/2  "MCU1_ActTMTorque"
  Subsystem/1(MCU1_TMSpeed) -> Bus Creator/1  "MCU1_TMSpeed"
  Bus Creator/1 -> Out1/1
  Subsystem/14(bool_MCUPwrDwnAllow) -> Bus Creator/14  "bool_MCUPwrDownAllow"

== system HQEV_MiL_20160830_integrate/MiL/Test_Integration/MCU_FF/MCU/MCU/Torque_Control ==
  In1 : Inport
  function : TriggerPort  TriggerType=function-call
  Bus Creator : BusCreator  Inputs=14
  Subsystem : Subsystem
  Out1 : Outport
  wires:
  In1/1 -> Subsystem/1(In1)
  Subsystem/3(MCU1_TMCapacitanceVoltage) -> Bus Creator/3  "MCU1_TMCapacitanceVoltage"
  Subsystem/1(MCU1_TMSpeed) -> Bus Creator/1  "MCU1_TMSpeed"
  Subsystem/4(MCU1_ActualTMTorqueValid) -> Bus Creator/4  "MCU1_ActualTMTorqueValid"
  Subsystem/5(MCU1_MCU1 PrechargeAllow) -> Bus Creator/5  "MCU1_MCU1 PrechargeAllow"
  Subsystem/6(MCU1_TMStatus) -> Bus Creator/6  "MCU1_TMStatus"
  Subsystem/7(MCU1_TMErrorStatus) -> Bus Creator/7  "MCU1_TMErrorStatus"
  Subsystem/8(MCU1_TM MAMTorque) -> Bus Creator/8  "MCU1_TMMAMTorque"
  Subsystem/9(MCU1_TM MAGTorque) -> Bus Creator/9  "MCU1_TMMAGTorque"
  Subsystem/11(MCU1_CoolingRequest) -> Bus Creator/11  "MCU1_CoolingRequest"
  Subsystem/12(PWM_Status) -> Bus Creator/12  "PWM_Status"
  Subsystem/13(EM_trq_req) -> Bus Creator/13  "EM_trq_req"
  Subsystem/14(bool_MCUPwrDwnAllow) -> Bus Creator/14  "bool_MCUPwrDownAllow"
  Bus Creator/1 -> Out1/1
  Subsystem/2(MCU1_ActTMTorque) -> Bus Creator/2  "MCU1_ActTMTorque"
  Subsystem/10(MCU1_CalTMTorque) -> Bus Creator/10  "MCU1_CalTMTorque"

== system HQEV_MiL_20160830_integrate/MiL/Test_Integration/MCU_FF/MCU/Signal/Checksum_MCU1_1 ==
  In1 : Inport
  Constant : Constant  Value=0
  Terminator : Terminator
  out : Outport
  wires:
  Constant/1 -> out/1
  In1/1 -> Terminator/1

== system HQEV_MiL_20160830_integrate/MiL/Test_Integration/MCU_FF/MCU/Signal/Checksum_MCU1_2 ==
  In1 : Inport
  Constant2 : Constant  Value=0
  Terminator : Terminator
  out : Outport
  wires:
  In1/1 -> Terminator/1
  Constant2/1 -> out/1

== system HQEV_MiL_20160830_integrate/MiL/Test_Integration/MCU_FF/MCU/Signal/LiveCounter_MCU1_1 ==
  In1 : Inport
  Constant : Constant  Value=0
  Terminator : Terminator
  out : Outport
  wires:
  Constant/1 -> out/1
  In1/1 -> Terminator/1

== system HQEV_MiL_20160830_integrate/MiL/Test_Integration/MCU_FF/MCU/Signal/LiveCounter_MCU1_2 ==
  In1 : Inport
  Constant : Constant  Value=0
  Terminator : Terminator
  out : Outport
  wires:
  Constant/1 -> out/1
  In1/1 -> Terminator/1

== system HQEV_MiL_20160830_integrate/MiL/Test_Integration/MCU_FF/MCU/Signal/MCU1_ActTMTorque ==
  In1 : Inport
  Bus Selector : BusSelector  OutputSignals=signal1.Motor_F.EM1_trq_out
  out : Outport
  wires:
  Bus Selector/1 -> out/1  "<EM1_trq_out>"
  In1/1 -> Bus Selector/1

== system HQEV_MiL_20160830_integrate/MiL/Test_Integration/MCU_FF/MCU/Signal/MCU1_ActualTMTorqueValid ==
  In1 : Inport
  Bus Selector : BusSelector  OutputSignals=signal2.MCU1_ActualTMTorqueValid
  out : Outport
  wires:
  In1/1 -> Bus Selector/1
  Bus Selector/1 -> out/1  "<MCU1_ActualTMTorqueValid>"

== system HQEV_MiL_20160830_integrate/MiL/Test_Integration/MCU_FF/MCU/Signal/MCU1_CalTMTorque ==
  In1 : Inport
  Bus Selector : BusSelector  OutputSignals=signal2.MCU1_CalTMTorque
  out : Outport
  wires:
  In1/1 -> Bus Selector/1
  Bus Selector/1 -> out/1  "<MCU1_CalTMTorque>"

== system HQEV_MiL_20160830_integrate/MiL/Test_Integration/MCU_FF/MCU/Signal/MCU1_CoolingRequest ==
  In1 : Inport
  Bus Selector : BusSelector  OutputSignals=signal2.MCU1_CoolingRequest
  out : Outport
  wires:
  In1/1 -> Bus Selector/1
  Bus Selector/1 -> out/1  "<MCU1_CoolingRequest>"

== system HQEV_MiL_20160830_integrate/MiL/Test_Integration/MCU_FF/MCU/Signal/MCU1_PrechargeAllow ==
  In1 : Inport
  Bus Selector : BusSelector  OutputSignals=signal2.MCU1_MCU1 PrechargeAllow
  out : Outport
  wires:
  In1/1 -> Bus Selector/1
  Bus Selector/1 -> out/1  "<MCU1_MCU1 PrechargeAllow>"

== system HQEV_MiL_20160830_integrate/MiL/Test_Integration/MCU_FF/MCU/Signal/MCU1_ShutdownEnable ==
  In1 : Inport
  Bus Selector : BusSelector  OutputSignals=signal2.bool_MCUPwrDownAllow
  out : Outport
  wires:
  Bus Selector/1 -> out/1  "<bool_MCUPwrDownAllow>"
  In1/1 -> Bus Selector/1

== system HQEV_MiL_20160830_integrate/MiL/Test_Integration/MCU_FF/MCU/Signal/MCU1_TMCapacitanceVoltage ==
  In1 : Inport
  Bus Selector : BusSelector  OutputSignals=signal1.Motor_F.EM1_U
  out : Outport
  wires:
  In1/1 -> Bus Selector/1
  Bus Selector/1 -> out/1  "<EM1_U>"

== system HQEV_MiL_20160830_integrate/MiL/Test_Integration/MCU_FF/MCU/Signal/MCU1_TMErrorStatus ==
  In1 : Inport
  Bus Selector : BusSelector  OutputSignals=signal2.MCU1_TMErrorStatus
  out : Outport
  wires:
  In1/1 -> Bus Selector/1
  Bus Selector/1 -> out/1  "<MCU1_TMErrorStatus>"

== system HQEV_MiL_20160830_integrate/MiL/Test_Integration/MCU_FF/MCU/Signal/MCU1_TMSpeed ==
  In1 : Inport
  Bus Selector : BusSelector  OutputSignals=signal1.Motor_F.EM1_spd
  out : Outport
  wires:
  In1/1 -> Bus Selector/1
  Bus Selector/1 -> out/1  "<EM1_spd>"

== system HQEV_MiL_20160830_integrate/MiL/Test_Integration/MCU_FF/MCU/Signal/MCU1_TMStatus ==
  In1 : Inport
  Bus Selector : BusSelector  OutputSignals=signal2.MCU1_TMStatus
  out : Outport
  wires:
  In1/1 -> Bus Selector/1
  Bus Selector/1 -> out/1  "<MCU1_TMStatus>"

== system HQEV_MiL_20160830_integrate/MiL/Test_Integration/MCU_FF/MCU/Signal/MCU1_TM_MAGTorque ==
  In1 : Inport
  Bus Selector : BusSelector  OutputSignals=signal2.MCU1_TMMAGTorque
  out : Outport
  wires:
  In1/1 -> Bus Selector/1
  Bus Selector/1 -> out/1  "<MCU1_TMMAGTorque>"

== system HQEV_MiL_20160830_integrate/MiL/Test_Integration/MCU_FF/MCU/Signal/MCU1_TM_MAMTorque ==
  In1 : Inport
  Bus Selector : BusSelector  OutputSignals=signal2.MCU1_TMMAMTorque
  out : Outport
  wires:
  In1/1 -> Bus Selector/1
  Bus Selector/1 -> out/1  "<MCU1_TMMAMTorque>"

== system HQEV_MiL_20160830_integrate/MiL/Test_Integration/MCU_FF/MCU/Signal/MCU1_trq_req ==
  In1 : Inport
  Bus Selector : BusSelector  OutputSignals=signal2.EM_trq_req
  out : Outport
  wires:
  In1/1 -> Bus Selector/1
  Bus Selector/1 -> out/1  "<EM_trq_req>"

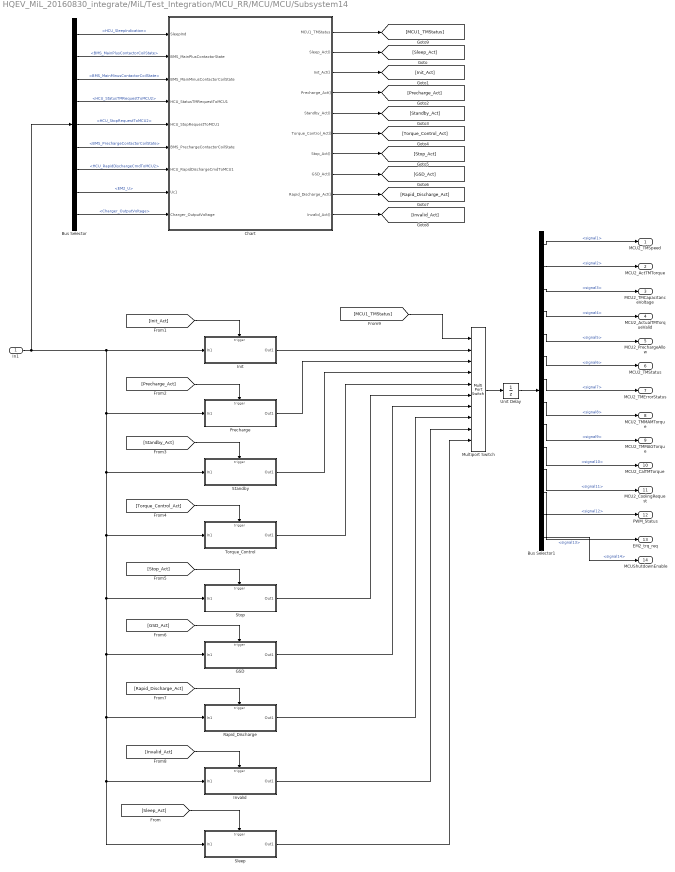
== system HQEV_MiL_20160830_integrate/MiL/Test_Integration/MCU_RR/MCU/MCU/Subsystem14 ==
  In1 : Inport
  Bus Selector : BusSelector  OutputSignals=HCU.HCU_SleepIndication,BMS.BMS_MainPlusContactorCoilState,BMS.BMS_MainMinusContactorCoilState,HCU.HCU_StatusTMRequestToMCU2,HCU.HCU_StopRequestToMCU2,BMS.BMS_PrechargeContactorCoilState,HCU.HCU_RapidDischargeCmdToMCU2,Motor_R.EM2_U,Charger.Charger_OutputVoltage
  Bus Selector1 : BusSelector  OutputSignals=signal1,signal2,signal3,signal4,signal5,signal6,signal7,signal8,signal9,signal10,signal11,signal12,signal13,signal14
  Chart : Stateflow chart  TreatAsAtomicUnit=on
  GSD : Subsystem  TreatAsAtomicUnit=on
  Init : Subsystem  TreatAsAtomicUnit=on
  Invalid : Subsystem  TreatAsAtomicUnit=on
  Multiport Switch : MultiPortSwitch  DataPortOrder=Zero-based contiguous  Inputs=9  zeroidx=on
  Precharge : Subsystem  TreatAsAtomicUnit=on
  Rapid_Discharge : Subsystem  TreatAsAtomicUnit=on
  Sleep : Subsystem  TreatAsAtomicUnit=on
  Standby : Subsystem  TreatAsAtomicUnit=on
  Stop : Subsystem  TreatAsAtomicUnit=on
  Torque_Control : Subsystem  TreatAsAtomicUnit=on
  Unit Delay : UnitDelay  SampleTime=-1
  MCU2_TMSpeed : Outport
  MCU2_ActTMTorque : Outport  Port=2
  MCU2_TMCapacitanceVoltage : Outport  Port=3
  MCU2_ActualTMTorqueValid : Outport  Port=4
  MCU2_PrechargeAllow : Outport  Port=5
  MCU2_TMStatus : Outport  Port=6
  MCU2_TMErrorStatus : Outport  Port=7
  MCU2_TMMAMTorque : Outport  Port=8
  MCU2_TMMAGTorque : Outport  Port=9
  MCU2_CalTMTorque : Outport  Port=10
  MCU2_CoolingRequest : Outport  Port=11
  PWM_Status : Outport  Port=12
  EM2_trq_req : Outport  Port=13
  MCUShutdownEnable : Outport  Port=14
  wires:
  Chart/2(Sleep_Act()) -> [Sleep_Act]
  Chart/3(Init_Act()) -> [Init_Act]
  Chart/4(Precharge_Act()) -> [Precharge_Act]
  Chart/5(Standby_Act()) -> [Standby_Act]
  Chart/6(Torque_Control_Act()) -> [Torque_Control_Act]
  Chart/7(Stop_Act()) -> [Stop_Act]
  Chart/8(GSD_Act()) -> [GSD_Act]
  Chart/9(Rapid_Discharge_Act()) -> [Rapid_Discharge_Act]
  Chart/10(Invalid_Act()) -> [Invalid_Act]
  Chart/1(MCU1_TMStatus) -> [MCU1_TMStatus]
  [Init_Act] -> Init/Trigger
  [Precharge_Act] -> Precharge/Trigger
  [Torque_Control_Act] -> Torque_Control/Trigger
  [Stop_Act] -> Stop/Trigger
  [Rapid_Discharge_Act] -> Rapid_Discharge/Trigger
  [Invalid_Act] -> Invalid/Trigger
  [Standby_Act] -> Standby/Trigger
  [GSD_Act] -> GSD/Trigger
  Init/1(Out1) -> Multiport Switch/2
  Precharge/1(Out1) -> Multiport Switch/3
  Standby/1(Out1) -> Multiport Switch/4
  Torque_Control/1(Out1) -> Multiport Switch/5
  Stop/1(Out1) -> Multiport Switch/6
  GSD/1(Out1) -> Multiport Switch/7
  Rapid_Discharge/1(Out1) -> Multiport Switch/8
  Invalid/1(Out1) -> Multiport Switch/9
  [Sleep_Act] -> Sleep/Trigger
  Sleep/1(Out1) -> Multiport Switch/10
  [MCU1_TMStatus] -> Multiport Switch/1
  In1/1 -> Init/1(In1), Precharge/1(In1), Standby/1(In1), Torque_Control/1(In1), Stop/1(In1), GSD/1(In1), Rapid_Discharge/1(In1), Invalid/1(In1), Sleep/1(In1), Bus Selector/1
  Multiport Switch/1 -> Unit Delay/1
  Bus Selector/1 -> Chart/1(SleepInd)  "<HCU_SleepIndication>"
  Bus Selector/2 -> Chart/2(BMS_MainPlusContactorState)  "<BMS_MainPlusContactorCoilState>"
  Bus Selector/3 -> Chart/3(BMS_MainMinusContactorCoilState)  "<BMS_MainMinusContactorCoilState>"
  Bus Selector/4 -> Chart/4(HCU_StatusTMRequestToMCU1)  "<HCU_StatusTMRequestToMCU2>"
  Bus Selector/5 -> Chart/5(HCU_StopRequestToMCU1)  "<HCU_StopRequestToMCU2>"
  Bus Selector/6 -> Chart/6(BMS_PrechargeContactorCoilState)  "<BMS_PrechargeContactorCoilState>"
  Bus Selector/7 -> Chart/7(HCU_RapidDischargeCmdToMCU1)  "<HCU_RapidDischargeCmdToMCU2>"
  Bus Selector/8 -> Chart/8(Uc1)  "<EM2_U>"
  Unit Delay/1 -> Bus Selector1/1
  Bus Selector1/1 -> MCU2_TMSpeed/1  "<signal1>"
  Bus Selector1/2 -> MCU2_ActTMTorque/1  "<signal2>"
  Bus Selector1/3 -> MCU2_TMCapacitanceVoltage/1  "<signal3>"
  Bus Selector1/4 -> MCU2_ActualTMTorqueValid/1  "<signal4>"
  Bus Selector1/5 -> MCU2_PrechargeAllow/1  "<signal5>"
  Bus Selector1/6 -> MCU2_TMStatus/1  "<signal6>"
  Bus Selector1/7 -> MCU2_TMErrorStatus/1  "<signal7>"
  Bus Selector1/8 -> MCU2_TMMAMTorque/1  "<signal8>"
  Bus Selector1/9 -> MCU2_TMMAGTorque/1  "<signal9>"
  Bus Selector1/10 -> MCU2_CalTMTorque/1  "<signal10>"
  Bus Selector1/11 -> MCU2_CoolingRequest/1  "<signal11>"
  Bus Selector1/12 -> PWM_Status/1  "<signal12>"
  Bus Selector1/13 -> EM2_trq_req/1  "<signal13>"
  Bus Selector/9 -> Chart/9(Charger_OutputVoltage)  "<Charger_OutputVoltage>"
  Bus Selector1/14 -> MCUShutdownEnable/1  "<signal14>"

== system HQEV_MiL_20160830_integrate/MiL/Test_Integration/MCU_RR/MCU/Signal/Checksum_MCU2_1 ==
  In1 : Inport
  Constant : Constant  Value=0
  Terminator : Terminator
  out : Outport
  wires:
  Constant/1 -> out/1
  In1/1 -> Terminator/1

== system HQEV_MiL_20160830_integrate/MiL/Test_Integration/MCU_RR/MCU/Signal/Checksum_MCU2_2 ==
  In1 : Inport
  Constant2 : Constant  Value=0
  Terminator : Terminator
  out : Outport
  wires:
  In1/1 -> Terminator/1
  Constant2/1 -> out/1

== system HQEV_MiL_20160830_integrate/MiL/Test_Integration/MCU_RR/MCU/Signal/LiveCounter_MCU2_1 ==
  In1 : Inport
  Constant : Constant  Value=0
  Terminator : Terminator
  out : Outport
  wires:
  Constant/1 -> out/1
  In1/1 -> Terminator/1

== system HQEV_MiL_20160830_integrate/MiL/Test_Integration/MCU_RR/MCU/Signal/LiveCounter_MCU2_2 ==
  In1 : Inport
  Constant : Constant  Value=0
  Terminator : Terminator
  out : Outport
  wires:
  Constant/1 -> out/1
  In1/1 -> Terminator/1

== system HQEV_MiL_20160830_integrate/MiL/Test_Integration/MCU_RR/MCU/Signal/MCU2_ActTMTorque ==
  In1 : Inport
  Bus Selector : BusSelector  OutputSignals=signal1.Motor_R.EM2_trq_out
  out : Outport
  wires:
  Bus Selector/1 -> out/1  "<EM2_trq_out>"
  In1/1 -> Bus Selector/1

== system HQEV_MiL_20160830_integrate/MiL/Test_Integration/MCU_RR/MCU/Signal/MCU2_ActualTMTorqueValid ==
  In1 : Inport
  Bus Selector : BusSelector  OutputSignals=signal2.MCU2_ActualTMTorqueValid
  out : Outport
  wires:
  In1/1 -> Bus Selector/1
  Bus Selector/1 -> out/1  "<MCU2_ActualTMTorqueValid>"

== system HQEV_MiL_20160830_integrate/MiL/Test_Integration/MCU_RR/MCU/Signal/MCU2_CalTMTorque ==
  In1 : Inport
  Bus Selector : BusSelector  OutputSignals=signal2.MCU2_CalTMTorque
  out : Outport
  wires:
  In1/1 -> Bus Selector/1
  Bus Selector/1 -> out/1  "<MCU2_CalTMTorque>"

== system HQEV_MiL_20160830_integrate/MiL/Test_Integration/MCU_RR/MCU/Signal/MCU2_CoolingRequest ==
  In1 : Inport
  Bus Selector : BusSelector  OutputSignals=signal2.MCU2_CoolingRequest
  out : Outport
  wires:
  In1/1 -> Bus Selector/1
  Bus Selector/1 -> out/1  "<MCU2_CoolingRequest>"

== system HQEV_MiL_20160830_integrate/MiL/Test_Integration/MCU_RR/MCU/Signal/MCU2_PrechargeAllow ==
  In1 : Inport
  Bus Selector : BusSelector  OutputSignals=signal2.MCU2_PrechargeAllow
  out : Outport
  wires:
  In1/1 -> Bus Selector/1
  Bus Selector/1 -> out/1  "<MCU2_PrechargeAllow>"

== system HQEV_MiL_20160830_integrate/MiL/Test_Integration/MCU_RR/MCU/Signal/MCU2_TMCapacitanceVoltage ==
  In1 : Inport
  Bus Selector : BusSelector  OutputSignals=signal1.Motor_R.EM2_U
  out : Outport
  wires:
  In1/1 -> Bus Selector/1
  Bus Selector/1 -> out/1  "<EM2_U>"

== system HQEV_MiL_20160830_integrate/MiL/Test_Integration/MCU_RR/MCU/Signal/MCU2_TMErrorStatus ==
  In1 : Inport
  Bus Selector : BusSelector  OutputSignals=signal2.MCU2_TMErrorStatus
  out : Outport
  wires:
  In1/1 -> Bus Selector/1
  Bus Selector/1 -> out/1  "<MCU2_TMErrorStatus>"

== system HQEV_MiL_20160830_integrate/MiL/Test_Integration/MCU_RR/MCU/Signal/MCU2_TMSpeed ==
  In1 : Inport
  Bus Selector : BusSelector  OutputSignals=signal1.Motor_R.EM2_spd
  out : Outport
  wires:
  In1/1 -> Bus Selector/1
  Bus Selector/1 -> out/1  "<EM2_spd>"

== system HQEV_MiL_20160830_integrate/MiL/Test_Integration/MCU_RR/MCU/Signal/MCU2_TMStatus ==
  In1 : Inport
  Bus Selector : BusSelector  OutputSignals=signal2.MCU2_TMStatus
  out : Outport
  wires:
  In1/1 -> Bus Selector/1
  Bus Selector/1 -> out/1  "<MCU2_TMStatus>"

== system HQEV_MiL_20160830_integrate/MiL/Test_Integration/MCU_RR/MCU/Signal/MCU2_TM_MAGTorque ==
  In1 : Inport
  Bus Selector : BusSelector  OutputSignals=signal2.MCU2_TMMAGTorque
  out : Outport
  wires:
  In1/1 -> Bus Selector/1
  Bus Selector/1 -> out/1  "<MCU2_TMMAGTorque>"
